simulink model "Ebike_Thermal_DT_v1"  (R2026a)
settings: configuration reference "VehicleVariable" (kept outside this file)
StartFcn:
  | %tic
StopFcn:
  | %toc
model workspace (MAT data in the model file):
  ExtDrvCmdsSwitch : Simulink.Parameter (value not decoded)
  ExtDrvRefSwitch : Simulink.Parameter (value not decoded)
  ExtEnvSwitch : Simulink.Parameter (value not decoded)
  ExtGndSwitch : Simulink.Parameter (value not decoded)
symbols that are objects in the model workspace (value not decoded): ExtDrvCmdsSwitch, ExtDrvRefSwitch, ExtEnvSwitch, ExtGndSwitch
undefined symbols (not defined in the file or in its folder): AmbTemp, BaroPress, CtrlTcuInitGear, CurvGradRef, CurvRef, DCM, DriverAeroRes, DriverDrivelineRes, DriverInitialGear, DriverPreviewDist, DriverRollRes, DriverShiftTime, DriverTimeConst, DriverTractiveForce, EnvAbsPrs, EnvAirTemp, EnvGrvty, EnvNomFrictionScaling, EnvNominalGrade, EnvScnFrictionMap, EnvScnFrictionMapXBpts, EnvScnFrictionMapYBpts, EnvScnHeightMap, EnvScnHeightMapXBpts, EnvScnHeightMapYBpts, EnvWindVelX, EnvWindVelY, EnvWindVelZ, Gnd, Grade, HazzardCmd, HighBeamCmd, lambda_mux, LeftSignalCmd, LngRef, LowBeamCmd, LtrRef, PhiRef, PlntThrCabRelHInit, PlntThrRefrigPinit, PlntVehDstCGRearAxl, PlntVehInitYawAng, PlntVehMass, PlntVehTrckWdth, PlntVehYawMomentInertia, PlntWhlLdRadiusFrnt, PlntWhlLdRadiusRear, PsiRef, RightSignalCmd, Sim3dSensor, Wind, XRef, YRef, Z
libraries: simulink x28, autolibutils x5, autolibsharedcommon x5, vehdynlibviscommon x4, vehdynlibdriver x2, sim3dgroundtruthsensorlib x2, autolibshared x2, sl3dlib x1, sharedtransform x1, sim3dlib x1
(part 5 of 5)

== system Ebike_Thermal_DT_v1/Environment/Varying Friction/Friction Map/2D Lookup Tbl for Scaling Fctr (Lambda) ==
  XWhl : Inport  Partition=on  PartitionDimension=1  PartitionWidth=1  PartitionOffset=0
  YWhl : Inport  Port=2  Partition=on  PartitionDimension=1  PartitionWidth=1  PartitionOffset=0
  2-D Lookup Table : Lookup_n-D  BreakpointsForDimension1=EnvScnFrictionMapXBpts  BreakpointsForDimension2=EnvScnFrictionMapYBpts  BeginIndexSearchUsingPreviousIndexResult=on  Table=EnvScnFrictionMap  InterpMethod=Nearest  ExtrapMethod=Clip  InternalRulePriority=Speed  RndMeth=Simplest
      settings: InputPortMap=u0,u1
  Add : Sum
  Add1 : Sum
  Constant : Constant  Value=0
  Constant1 : Constant  Value=0
  For Each : ForEach  DisableCoverage=on
  Unary Minus : UnaryMinus
  FricCoeffLambda : Outport  ConcatenationDimension=1
  wires:
  2-D Lookup Table/1 -> FricCoeffLambda/1
  YWhl/1 -> Unary Minus/1
  Constant1/1 -> Add1/1
  Constant/1 -> Add/2
  Add/1 -> 2-D Lookup Table/2
  Add1/1 -> 2-D Lookup Table/1
  Unary Minus/1 -> Add/1
  XWhl/1 -> Add1/2

== system Ebike_Thermal_DT_v1/Environment/Varying Friction/Friction Map/Wheel Coordinates ==
  FrntAxlLftX : Inport
  FrntAxlRghtX : Inport  Port=2
  RearAxlLftX : Inport  Port=3
  RearAxlRghtX : Inport  Port=4
  FrntAxlLftY : Inport  Port=5
  FrntAxlRghtY : Inport  Port=6
  RearAxlLftY : Inport  Port=7
  RearAxlRghtY : Inport  Port=8
  Matrix Concatenate : Concatenate  NumInputs=4  Mode=Multidimensional array
  Matrix Concatenate1 : Concatenate  NumInputs=4  Mode=Multidimensional array
  XWhl : Outport
  YWhl : Outport  Port=2
  wires:
  Matrix Concatenate1/1 -> YWhl/1
  FrntAxlLftX/1 -> Matrix Concatenate/1
  FrntAxlLftY/1 -> Matrix Concatenate1/1
  FrntAxlRghtY/1 -> Matrix Concatenate1/2
  FrntAxlRghtX/1 -> Matrix Concatenate/2
  RearAxlLftY/1 -> Matrix Concatenate1/3
  RearAxlLftX/1 -> Matrix Concatenate/3
  RearAxlRghtY/1 -> Matrix Concatenate1/4
  Matrix Concatenate/1 -> XWhl/1
  RearAxlRghtX/1 -> Matrix Concatenate/4

== system Ebike_Thermal_DT_v1/Environment/Varying Friction/Varying Friction/Road Track Friction ==
  XWhl : Inport
  YWhl : Inport  Port=2
  Cg : Inport  Port=3
  2D Lookup Tbl for Scaling Fctr (Lambda) : Subsystem  TreatAsAtomicUnit=on
      mask init:
      | [~]=vehdynicon('vehdynblk',gcb);
  Bus Selector : BusSelector  OutputSignals=X,Y
  Cnst Lambda : Constant  Value=ones(4,1).*lambda_g
  Constant1 : Constant  Value=SplitLambdaTrck
  Creating Inertial Frm Bpt : Subsystem
  En at t = 0 : Subsystem
  "Lambda (t = 0) " : Memory  InitialCondition=ones(4,1).*lambda_g  InheritSampleTime=on
  Switch : Switch  Criteria=u2 > Threshold  SaturateOnIntegerOverflow=off  InputSameDT=off
  FricCoeffLambda : Outport
  wires:
  YWhl/1 -> 2D Lookup Tbl for Scaling Fctr (Lambda)/2(YWhl)
  XWhl/1 -> 2D Lookup Tbl for Scaling Fctr (Lambda)/1(XWhl)
  2D Lookup Tbl for Scaling Fctr (Lambda)/1(Lambda for each whl) -> Switch/1
  "Lambda (t = 0) "/1 -> FricCoeffLambda/1
  Switch/1 -> "Lambda (t = 0) "/1
  Cnst Lambda/1 -> Switch/3
  Constant1/1 -> Switch/2
  Cg/1 -> Bus Selector/1
  Creating Inertial Frm Bpt/1(XBpt) -> 2D Lookup Tbl for Scaling Fctr (Lambda)/3(XBpt)
  Creating Inertial Frm Bpt/2(YBpt) -> 2D Lookup Tbl for Scaling Fctr (Lambda)/4(YBpt)
  Bus Selector/1 -> Creating Inertial Frm Bpt/1(XCg)  "<X>"
  Bus Selector/2 -> Creating Inertial Frm Bpt/2(YCg)  "<Y>"
  En at t = 0/1(Out1) -> Creating Inertial Frm Bpt/Enable

== system Ebike_Thermal_DT_v1/Environment/Varying Friction/Varying Friction/Wheel Coordinates ==
  FrntAxlLftX : Inport
  FrntAxlRghtX : Inport  Port=2
  RearAxlLftX : Inport  Port=3
  RearAxlRghtX : Inport  Port=4
  FrntAxlLftY : Inport  Port=5
  FrntAxlRghtY : Inport  Port=6
  RearAxlLftY : Inport  Port=7
  RearAxlRghtY : Inport  Port=8
  Matrix Concatenate : Concatenate  NumInputs=4  Mode=Multidimensional array
  Matrix Concatenate1 : Concatenate  NumInputs=4  Mode=Multidimensional array
  XWhl : Outport
  YWhl : Outport  Port=2
  wires:
  RearAxlRghtX/1 -> Matrix Concatenate/4
  Matrix Concatenate/1 -> XWhl/1
  RearAxlRghtY/1 -> Matrix Concatenate1/4
  RearAxlLftX/1 -> Matrix Concatenate/3
  RearAxlLftY/1 -> Matrix Concatenate1/3
  FrntAxlRghtX/1 -> Matrix Concatenate/2
  FrntAxlRghtY/1 -> Matrix Concatenate1/2
  FrntAxlLftY/1 -> Matrix Concatenate1/1
  FrntAxlLftX/1 -> Matrix Concatenate/1
  Matrix Concatenate1/1 -> YWhl/1

== system Ebike_Thermal_DT_v1/Visualization/Vehicle XY Plotter/XY View/Driveline Speed ==
  <EngSpd> : Inport
  <EMSpd> : Inport  Port=2
  Abs : Abs  ZeroCross=off  SaturateOnIntegerOverflow=off
  Abs1 : Abs  ZeroCross=off  SaturateOnIntegerOverflow=off
  Divide : Product  Inputs=*/
  Probe Dimension : Probe  ProbeWidth=off  ProbeSampleTime=off  ProbeComplexSignal=off  ProbeSignalDimensions=on
  Relational Operator : RelationalOperator  Operator=<=  OutDataTypeStr=boolean  ZeroCross=off  RndMeth=Simplest  InputSameDT=off
  Sum of Elements : Sum  Inputs=+
  Switch : Switch  Criteria=u2 > Threshold  ZeroCross=off  SaturateOnIntegerOverflow=off  InputSameDT=off
  MaxSpd : Outport
  wires:
  Switch/1 -> MaxSpd/1
  Sum of Elements/1 -> Divide/1
  Probe Dimension/1 -> Divide/2
  Divide/1 -> Switch/3, Abs1/1
  <EngSpd>/1 -> Switch/1, Abs/1
  Abs/1 -> Relational Operator/2
  <EMSpd>/1 -> Probe Dimension/1, Sum of Elements/1
  Relational Operator/1 -> Switch/2
  Abs1/1 -> Relational Operator/1

== system Ebike_Thermal_DT_v1/Visualization/Vehicle XY Plotter/XY View Ref/Driveline Speed ==
  <EngSpd> : Inport
  <EMSpd> : Inport  Port=2
  Abs : Abs  ZeroCross=off  SaturateOnIntegerOverflow=off
  Abs1 : Abs  ZeroCross=off  SaturateOnIntegerOverflow=off
  Divide : Product  Inputs=*/
  Probe Dimension : Probe  ProbeWidth=off  ProbeSampleTime=off  ProbeComplexSignal=off  ProbeSignalDimensions=on
  Relational Operator : RelationalOperator  Operator=<=  OutDataTypeStr=boolean  ZeroCross=off  RndMeth=Simplest  InputSameDT=off
  Sum of Elements : Sum  Inputs=+
  Switch : Switch  Criteria=u2 > Threshold  ZeroCross=off  SaturateOnIntegerOverflow=off  InputSameDT=off
  MaxSpd : Outport
  wires:
  Switch/1 -> MaxSpd/1
  Sum of Elements/1 -> Divide/1
  Probe Dimension/1 -> Divide/2
  Divide/1 -> Switch/3, Abs1/1
  <EngSpd>/1 -> Switch/1, Abs/1
  Abs/1 -> Relational Operator/2
  <EMSpd>/1 -> Probe Dimension/1, Sum of Elements/1
  Relational Operator/1 -> Switch/2
  Abs1/1 -> Relational Operator/1

== system Ebike_Thermal_DT_v1/Visualization/Vehicle XY Plotter/XY View Ref with One-Axle Trailer/Driveline Speed ==
  <EngSpd> : Inport
  <EMSpd> : Inport  Port=2
  Abs : Abs  ZeroCross=off  SaturateOnIntegerOverflow=off
  Abs1 : Abs  ZeroCross=off  SaturateOnIntegerOverflow=off
  Divide : Product  Inputs=*/
  Probe Dimension : Probe  ProbeWidth=off  ProbeSampleTime=off  ProbeComplexSignal=off  ProbeSignalDimensions=on
  Relational Operator : RelationalOperator  Operator=<=  OutDataTypeStr=boolean  ZeroCross=off  RndMeth=Simplest  InputSameDT=off
  Sum of Elements : Sum  Inputs=+
  Switch : Switch  Criteria=u2 > Threshold  ZeroCross=off  SaturateOnIntegerOverflow=off  InputSameDT=off
  MaxSpd : Outport
  wires:
  Switch/1 -> MaxSpd/1
  Sum of Elements/1 -> Divide/1
  Probe Dimension/1 -> Divide/2
  Divide/1 -> Switch/3, Abs1/1
  <EngSpd>/1 -> Switch/1, Abs/1
  Abs/1 -> Relational Operator/2
  <EMSpd>/1 -> Probe Dimension/1, Sum of Elements/1
  Relational Operator/1 -> Switch/2
  Abs1/1 -> Relational Operator/1

== system Ebike_Thermal_DT_v1/Driver Commands/Driver Commands/Longitudinal Driver/Hill Hold & Stop/Hill Hold ==
  <EngSpdOut> : Inport
  <xdot> : Inport  Port=2
  <BattSoc> : Inport  Port=3
  LngRef : Inport  Port=4
  <Grade> : Inport  Port=5
  Abs : Abs  ZeroCross=off  SaturateOnIntegerOverflow=off
  Abs1 : Abs  ZeroCross=off  SaturateOnIntegerOverflow=off
  Compare To Constant : simulink/Logic and Bit Operations/Compare To Constant  relop=<=  const=.1  OutDataTypeStr=boolean  ZeroCross=off
  Compare To Constant1 : simulink/Logic and Bit Operations/Compare To Constant  relop=>=  const=.1  OutDataTypeStr=boolean  ZeroCross=off
  Compare To Constant2 : simulink/Logic and Bit Operations/Compare To Constant  relop=<=  const=500  OutDataTypeStr=boolean  ZeroCross=off
  Compare To Constant3 : simulink/Logic and Bit Operations/Compare To Constant  relop=<=  const=5  OutDataTypeStr=boolean  ZeroCross=off
  Compare To Constant4 : simulink/Logic and Bit Operations/Compare To Constant  relop=<=  const=.1  OutDataTypeStr=boolean  ZeroCross=off
  Data Type Conversion1 : DataTypeConversion  SaturateOnIntegerOverflow=off  RndMeth=Floor
  Logical Operator : Logic  AllPortsSameDT=off  OutDataTypeStr=boolean
  Logical Operator1 : Logic  Inputs=3  AllPortsSameDT=off  OutDataTypeStr=boolean
  Logical Operator2 : Logic  Operator=OR  AllPortsSameDT=off  OutDataTypeStr=boolean
  Signal Specification : SignalSpecification  Unit=m/s
  Unit Conversion : UnitConversion
  DecelOvr : Outport
  EnblDecelOvr : Outport  Port=2
  wires:
  <BattSoc>/1 -> Compare To Constant4/1
  <xdot>/1 -> Unit Conversion/1
  <Grade>/1 -> Abs1/1
  Compare To Constant4/1 -> Logical Operator1/3
  <EngSpdOut>/1 -> Compare To Constant2/1
  Signal Specification/1 -> Compare To Constant3/1
  Abs/1 -> Compare To Constant/1
  Logical Operator1/1 -> Logical Operator2/1
  Data Type Conversion1/1 -> EnblDecelOvr/1
  Compare To Constant2/1 -> Logical Operator1/1
  Logical Operator/1 -> Logical Operator2/2
  Compare To Constant3/1 -> Logical Operator1/2
  Compare To Constant1/1 -> Logical Operator/2
  LngRef/1 -> Abs/1
  Abs1/1 -> Compare To Constant1/1
  Logical Operator2/1 -> Data Type Conversion1/1, DecelOvr/1
  Unit Conversion/1 -> Signal Specification/1
  Compare To Constant/1 -> Logical Operator/1

== system Ebike_Thermal_DT_v1/Driver Commands/Driver Commands/Longitudinal Driver/Hill Hold & Stop/Stop Detection ==
  LngRef : Inport
  <xdot> : Inport  Port=2
  Abs2 : Abs  ZeroCross=off  SaturateOnIntegerOverflow=off
  Compare To Constant5 : simulink/Logic and Bit Operations/Compare To Constant  relop=<=  const=.1  OutDataTypeStr=boolean  ZeroCross=off
  Compare To Constant6 : simulink/Logic and Bit Operations/Compare To Constant  relop===  const=0  OutDataTypeStr=boolean  ZeroCross=off
  Data Type Conversion2 : DataTypeConversion  SaturateOnIntegerOverflow=off  RndMeth=Floor
  Gain : Gain  Gain=.1
  LatchSwitchCont : autolibutils/LatchSwitchCont  aMode=6
  Logical Operator1 : Logic  Operator=NOT  AllPortsSameDT=off  OutDataTypeStr=boolean
  Logical Operator3 : Logic  AllPortsSameDT=off  OutDataTypeStr=boolean
  DecelOvrCmd : Outport
  EnblDecelOvr : Outport  Port=2
  wires:
  <xdot>/1 -> Abs2/1
  Gain/1 -> DecelOvrCmd/1
  Compare To Constant6/1 -> Logical Operator3/2, Logical Operator1/1
  Logical Operator1/1 -> LatchSwitchCont/2
  Data Type Conversion2/1 -> Gain/1
  LatchSwitchCont/1 -> Data Type Conversion2/1, EnblDecelOvr/1
  Abs2/1 -> Compare To Constant5/1
  LngRef/1 -> Compare To Constant6/1
  Logical Operator3/1 -> LatchSwitchCont/1
  Compare To Constant5/1 -> Logical Operator3/1

== system Ebike_Thermal_DT_v1/Driver Commands/Driver Commands/Longitudinal Driver/Longitudinal Driver/External Action Routing ==
  EnblAccelOvr : Inport  OutDataTypeStr=boolean  Unit=1  PortDimensions=1
  AccelOvrCmd : Inport  Port=2  OutDataTypeStr=double  Unit=1  PortDimensions=1
  AccelHld : Inport  Port=3  OutDataTypeStr=boolean  Unit=1  PortDimensions=1
  AccelZero : Inport  Port=4  OutDataTypeStr=boolean  Unit=1  PortDimensions=1
  EnblDecelOvr : Inport  Port=5  OutDataTypeStr=boolean  Unit=1  PortDimensions=1
  DecelOvrCmd : Inport  Port=6  OutDataTypeStr=double  Unit=1  PortDimensions=1
  DecelHld : Inport  Port=7  OutDataTypeStr=boolean  Unit=1  PortDimensions=1
  DecelZero : Inport  Port=8  OutDataTypeStr=boolean  Unit=1  PortDimensions=1
  Bus Creator2 : BusCreator  Inputs=8
  ExtActions : Outport
  wires:
  Bus Creator2/1 -> ExtActions/1  "ExtActions"
  DecelZero/1 -> Bus Creator2/8  "DecelZero"
  DecelHld/1 -> Bus Creator2/7  "DecelHld"
  DecelOvrCmd/1 -> Bus Creator2/6  "DecelOvrCmd"
  EnblDecelOvr/1 -> Bus Creator2/5  "EnblDecelOvr"
  AccelZero/1 -> Bus Creator2/4  "AccelZero"
  AccelHld/1 -> Bus Creator2/3  "AccelHld"
  AccelOvrCmd/1 -> Bus Creator2/2  "AccelOvrCmd"
  EnblAccelOvr/1 -> Bus Creator2/1  "EnblAccelOvr"

== system Ebike_Thermal_DT_v1/Driver Commands/Driver Commands/Predictive Driver/Hill Hold & Stop/Hill Hold ==
  <EngSpdOut> : Inport
  <xdot> : Inport  Port=2
  <BattSoc> : Inport  Port=3
  LngRef : Inport  Port=4
  <Grade> : Inport  Port=5
  Abs : Abs  ZeroCross=off  SaturateOnIntegerOverflow=off
  Abs1 : Abs  ZeroCross=off  SaturateOnIntegerOverflow=off
  Compare To Constant : simulink/Logic and Bit Operations/Compare To Constant  relop=<=  const=.1  OutDataTypeStr=boolean  ZeroCross=off
  Compare To Constant1 : simulink/Logic and Bit Operations/Compare To Constant  relop=>=  const=.1  OutDataTypeStr=boolean  ZeroCross=off
  Compare To Constant2 : simulink/Logic and Bit Operations/Compare To Constant  relop=<=  const=500  OutDataTypeStr=boolean  ZeroCross=off
  Compare To Constant3 : simulink/Logic and Bit Operations/Compare To Constant  relop=<=  const=5  OutDataTypeStr=boolean  ZeroCross=off
  Compare To Constant4 : simulink/Logic and Bit Operations/Compare To Constant  relop=<=  const=.1  OutDataTypeStr=boolean  ZeroCross=off
  Data Type Conversion1 : DataTypeConversion  SaturateOnIntegerOverflow=off  RndMeth=Floor
  Logical Operator : Logic  AllPortsSameDT=off  OutDataTypeStr=boolean
  Logical Operator1 : Logic  Inputs=3  AllPortsSameDT=off  OutDataTypeStr=boolean
  Logical Operator2 : Logic  Operator=OR  AllPortsSameDT=off  OutDataTypeStr=boolean
  Signal Specification : SignalSpecification  Unit=m/s
  Unit Conversion : UnitConversion
  DecelOvr : Outport
  EnblDecelOvr : Outport  Port=2
  wires:
  <BattSoc>/1 -> Compare To Constant4/1
  <xdot>/1 -> Unit Conversion/1
  <Grade>/1 -> Abs1/1
  Compare To Constant4/1 -> Logical Operator1/3
  <EngSpdOut>/1 -> Compare To Constant2/1
  Signal Specification/1 -> Compare To Constant3/1
  Abs/1 -> Compare To Constant/1
  Logical Operator1/1 -> Logical Operator2/1
  Data Type Conversion1/1 -> EnblDecelOvr/1
  Compare To Constant2/1 -> Logical Operator1/1
  Logical Operator/1 -> Logical Operator2/2
  Compare To Constant3/1 -> Logical Operator1/2
  Compare To Constant1/1 -> Logical Operator/2
  LngRef/1 -> Abs/1
  Abs1/1 -> Compare To Constant1/1
  Logical Operator2/1 -> Data Type Conversion1/1, DecelOvr/1
  Unit Conversion/1 -> Signal Specification/1
  Compare To Constant/1 -> Logical Operator/1

== system Ebike_Thermal_DT_v1/Driver Commands/Driver Commands/Predictive Driver/Hill Hold & Stop/Stop Detection ==
  LngRef : Inport
  <xdot> : Inport  Port=2
  Abs2 : Abs  ZeroCross=off  SaturateOnIntegerOverflow=off
  Compare To Constant5 : simulink/Logic and Bit Operations/Compare To Constant  relop=<=  const=.1  OutDataTypeStr=boolean  ZeroCross=off
  Compare To Constant6 : simulink/Logic and Bit Operations/Compare To Constant  relop===  const=0  OutDataTypeStr=boolean  ZeroCross=off
  Data Type Conversion2 : DataTypeConversion  SaturateOnIntegerOverflow=off  RndMeth=Floor
  Gain : Gain  Gain=.1
  LatchSwitchCont : autolibutils/LatchSwitchCont  aMode=6
  Logical Operator1 : Logic  Operator=NOT  AllPortsSameDT=off  OutDataTypeStr=boolean
  Logical Operator3 : Logic  AllPortsSameDT=off  OutDataTypeStr=boolean
  DecelOvrCmd : Outport
  EnblDecelOvr : Outport  Port=2
  wires:
  <xdot>/1 -> Abs2/1
  Gain/1 -> DecelOvrCmd/1
  Compare To Constant6/1 -> Logical Operator3/2, Logical Operator1/1
  Logical Operator1/1 -> LatchSwitchCont/2
  Data Type Conversion2/1 -> Gain/1
  LatchSwitchCont/1 -> Data Type Conversion2/1, EnblDecelOvr/1
  Abs2/1 -> Compare To Constant5/1
  LngRef/1 -> Compare To Constant6/1
  Logical Operator3/1 -> LatchSwitchCont/1
  Compare To Constant5/1 -> Logical Operator3/1

== system Ebike_Thermal_DT_v1/Driver Commands/Driver Commands/Predictive Stanley Driver/Hill Hold & Stop/Hill Hold ==
  <EngSpdOut> : Inport
  <xdot> : Inport  Port=2
  <BattSoc> : Inport  Port=3
  LngRef : Inport  Port=4
  <Grade> : Inport  Port=5
  Abs : Abs  ZeroCross=off  SaturateOnIntegerOverflow=off
  Abs1 : Abs  ZeroCross=off  SaturateOnIntegerOverflow=off
  Compare To Constant : simulink/Logic and Bit Operations/Compare To Constant  relop=<=  const=.1  OutDataTypeStr=boolean  ZeroCross=off
  Compare To Constant1 : simulink/Logic and Bit Operations/Compare To Constant  relop=>=  const=.1  OutDataTypeStr=boolean  ZeroCross=off
  Compare To Constant2 : simulink/Logic and Bit Operations/Compare To Constant  relop=<=  const=500  OutDataTypeStr=boolean  ZeroCross=off
  Compare To Constant3 : simulink/Logic and Bit Operations/Compare To Constant  relop=<=  const=5  OutDataTypeStr=boolean  ZeroCross=off
  Compare To Constant4 : simulink/Logic and Bit Operations/Compare To Constant  relop=<=  const=.1  OutDataTypeStr=boolean  ZeroCross=off
  Data Type Conversion1 : DataTypeConversion  SaturateOnIntegerOverflow=off  RndMeth=Floor
  Logical Operator : Logic  AllPortsSameDT=off  OutDataTypeStr=boolean
  Logical Operator1 : Logic  Inputs=3  AllPortsSameDT=off  OutDataTypeStr=boolean
  Logical Operator2 : Logic  Operator=OR  AllPortsSameDT=off  OutDataTypeStr=boolean
  Signal Specification : SignalSpecification  Unit=m/s
  Unit Conversion : UnitConversion
  DecelOvr : Outport
  EnblDecelOvr : Outport  Port=2
  wires:
  <BattSoc>/1 -> Compare To Constant4/1
  <xdot>/1 -> Unit Conversion/1
  <Grade>/1 -> Abs1/1
  Compare To Constant4/1 -> Logical Operator1/3
  <EngSpdOut>/1 -> Compare To Constant2/1
  Signal Specification/1 -> Compare To Constant3/1
  Abs/1 -> Compare To Constant/1
  Logical Operator1/1 -> Logical Operator2/1
  Data Type Conversion1/1 -> EnblDecelOvr/1
  Compare To Constant2/1 -> Logical Operator1/1
  Logical Operator/1 -> Logical Operator2/2
  Compare To Constant3/1 -> Logical Operator1/2
  Compare To Constant1/1 -> Logical Operator/2
  LngRef/1 -> Abs/1
  Abs1/1 -> Compare To Constant1/1
  Logical Operator2/1 -> Data Type Conversion1/1, DecelOvr/1
  Unit Conversion/1 -> Signal Specification/1
  Compare To Constant/1 -> Logical Operator/1

== system Ebike_Thermal_DT_v1/Driver Commands/Driver Commands/Predictive Stanley Driver/Hill Hold & Stop/Stop Detection ==
  LngRef : Inport
  <xdot> : Inport  Port=2
  Abs2 : Abs  ZeroCross=off  SaturateOnIntegerOverflow=off
  Compare To Constant5 : simulink/Logic and Bit Operations/Compare To Constant  relop=<=  const=.1  OutDataTypeStr=boolean  ZeroCross=off
  Compare To Constant6 : simulink/Logic and Bit Operations/Compare To Constant  relop===  const=0  OutDataTypeStr=boolean  ZeroCross=off
  Data Type Conversion2 : DataTypeConversion  SaturateOnIntegerOverflow=off  RndMeth=Floor
  Gain : Gain  Gain=.1
  LatchSwitchCont : autolibutils/LatchSwitchCont  aMode=6
  Logical Operator1 : Logic  Operator=NOT  AllPortsSameDT=off  OutDataTypeStr=boolean
  Logical Operator3 : Logic  AllPortsSameDT=off  OutDataTypeStr=boolean
  DecelOvrCmd : Outport
  EnblDecelOvr : Outport  Port=2
  wires:
  <xdot>/1 -> Abs2/1
  Gain/1 -> DecelOvrCmd/1
  Compare To Constant6/1 -> Logical Operator3/2, Logical Operator1/1
  Logical Operator1/1 -> LatchSwitchCont/2
  Data Type Conversion2/1 -> Gain/1
  LatchSwitchCont/1 -> Data Type Conversion2/1, EnblDecelOvr/1
  Abs2/1 -> Compare To Constant5/1
  LngRef/1 -> Compare To Constant6/1
  Logical Operator3/1 -> LatchSwitchCont/1
  Compare To Constant5/1 -> Logical Operator3/1

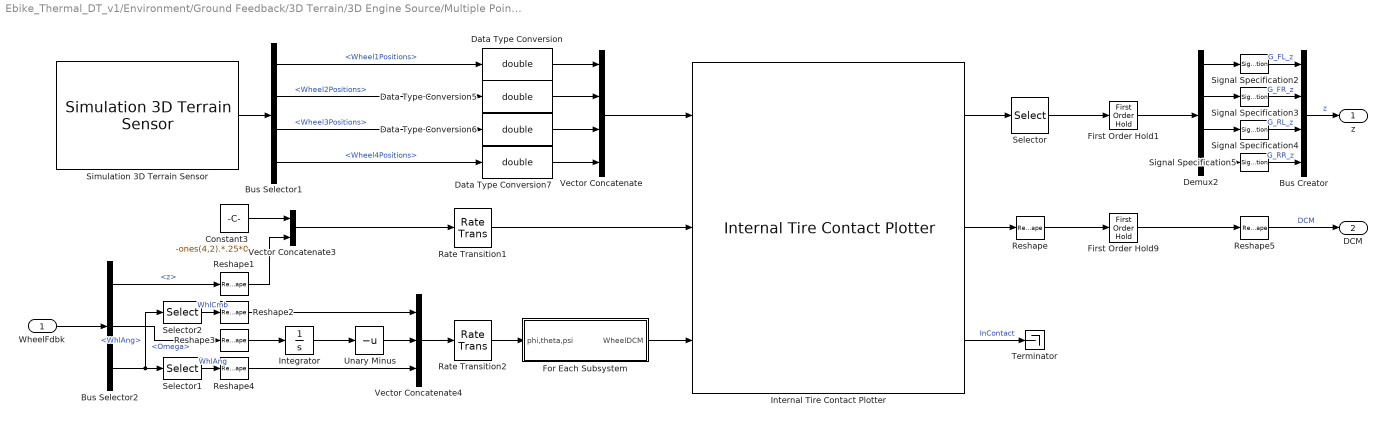
== system Ebike_Thermal_DT_v1/Environment/Ground Feedback/3D Terrain/3D Engine Source/Multiple Points ==
  WheelFdbk : Inport
  Bus Creator : BusCreator  Inputs=4
  Bus Selector1 : BusSelector  OutputSignals=Wheel1Positions,Wheel2Positions,Wheel3Positions,Wheel4Positions
  Bus Selector2 : BusSelector  OutputSignals=z,Omega,WhlAng
  Constant3 : Constant  Value=-ones(4,2).*.25*0
  Data Type Conversion{,5..7} (4 alike) : DataTypeConversion  OutDataTypeStr=double  SaturateOnIntegerOverflow=off  RndMeth=Floor
  Demux2 : Demux
  First Order Hold1 : FirstOrderHold  OutputAlgorithm=Fast (Minimize Error)  ErrorTolerance=.001
  First Order Hold9 : FirstOrderHold  InitialOutput=reshape(repmat(eye(3),1,1,4),[],1)  OutputAlgorithm=Fast (Minimize Error)  ErrorTolerance=.001
  For Each Subsystem : Subsystem  TreatAsAtomicUnit=on
  Integrator : Integrator  WrapState=on  ZeroCross=off
  Internal Tire Contact Plotter : vehdynlibviscommon/Internal Tire Contact Plotter  dispFig=off  numAxles=2  numWheelsPerAxle=2  wheelRad=.33  wheelWidth=.235  rayOrigins=[0.5 -0.5 0;0.4 -0.5 0;0.3 -0.5 0;0.19999999999999996 -0.5 0;0.099999999999999978 -0.5 0;0 -0.5 0;-0.099999999999999978 -0.5 0;-0.19999999999999996 -0.5 0;-0.3 -0.5 0;-0.4 -0.5 0;-0.5 -0.5 0;0.5 -0.4 0;0.4 -0.4 0;0.3 -0.4 0;0.19999999999999996 -0.4 0;0.099999999999999978 -0.4 0;0 -0.4 0;-0.099999999999999978 -0.4 0;-0.19999999999999996 -0.4 0;-0.3 -0.4 0;-0.4 -0.4 0;-0.5 -0.4 0;0.5 -0.3 0;0.4 -0.3 0;0.3 -0.3 0;0.19999999999999996 -0.3 0;0.099999999999999978 -0.3 0;0 -0.3 0;-0.099999999999999978 -0.3 0;-0.19999999999999996 -0.3 0;-0.3 -0.3 0;-0.4 -0.3 0;-0.5 -0.3 0;0.5 -0.19999999999999996 0;0.4 -0.19999999999999996 0;0.3 -0.19999999999999996 0;0.19999999999999996 -0.19999999999999996 0;0.099999999999999978 -0.19999999999999996 0;0 -0.19999999999999996 0;-0.099999999999999978 -0.19999999999999996 0;-0.19999999999999996 -0.19999999999999996 0;-0.3 -0.19999999999999996 0;-0.4 -0.19999999999999996 0;-0.5 -0.19999999999999996 0;0.5 -0.099999999999999978 0;0.4 -0.099999999999999978 0;0.3 -0.099999999999999978 0;0.19999999999999996 -0.099999999999999978 0;0.099999999999999978 -0.099999999999999978 0;0 -0.099999999999999978 0;-0.099999999999999978 -0.099999999999999978 0;-0.19999999999999996 -0.099999999999999978 0;-0.3 -0.099999999999999978 0;-0.4 -0.099999999999999978 0;-0.5 -0.099999999999999978 0;0.5 0 0;0.4 0 0;0.3 0 0;0.19999999999999996 0 0;0.099999999999999978 0 0;0 0 0;-0.099999999999999978 0 0;-0.19999999999999996 0 0;-0.3 0 0;-0.4 0 0;-0.5 0 0;0.5 0.099999999999999978 0;0.4 0.099999999999999978 0;0.3 0.099999999999999978 0;0.19999999999999996 0.099999999999999978 0;0.099999999999999978 0.099999999999999978 0;0 0.099999999999999978 0;-0.099999999999999978 0.099999999999999978 0;-0.19999999999999996 0.099999999999999978 0;-0.3 0.099999999999999978 0;-0.4 0.099999999999999978 0;-0.5 0.099999999999999978 0;0.5 0.19999999999999996 0;0.4 0.19999999999999996 0;0.3 0.19999999999999996 0;0.19999999999999996 0.19999999999999996 0;0.099999999999999978 0.19999999999999996 0;0 0.19999999999999996 0;-0.099999999999999978 0.19999999999999996 0;-0.19999999999999996 0.19999999999999996 0;-0.3 0.19999999999999996 0;-0.4 0.19999999999999996 0;-0.5 0.19999999999999996 0;0.5 0.3 0;0.4 0.3 0;0.3 0.3 0;0.19999999999999996 0.3 0;0.099999999999999978 0.3 0;0 0.3 0;-0.099999999999999978 0.3 0;-0.19999999999999996 0.3 0;-0.3 0.3 0;-0.4 0.3 0;-0.5 0.3 0;0.5 0.4 0;0.4 0.4 0;0.3 0.4 0;0.19999999999999996 0.4 0;0.099999999999999978 0.4 0;0 0.4 0;-0.099999999999999978 0.4 0;-0.19999999999999996 0.4 0;-0.3 0.4 0;-0.4 0.4 0;-0.5 0.4 0;0.5 0.5 0;0.4 0.5 0;0.3 0.5 0;0.19999999999999996 0.5 0;0.099999999999999978 0.5 0;0 0.5 0;-0.099999999999999978 0.5 0;-0.19999999999999996 0.5 0;-0.3 0.5 0;-0.4 0.5 0;-0.5 0.5 0]
  Rate Transition1 : RateTransition  Integrity=off  Deterministic=off  OutPortSampleTime=.01
  Rate Transition2 : RateTransition  Integrity=off  Deterministic=off  OutPortSampleTime=.01
  Reshape : Reshape  OutputDimensionality=Column vector (2-D)
  Reshape1 : Reshape  OutputDimensionality=Column vector (2-D)
  Reshape2 : Reshape  OutputDimensionality=Row vector (2-D)
  Reshape3 : Reshape  OutputDimensionality=Row vector (2-D)
  Reshape4 : Reshape  OutputDimensionality=Row vector (2-D)
  Reshape5 : Reshape  OutputDimensionality=Customize  OutputDimensions=[3,3,4]
  Selector : Selector  NumberOfDimensions=2  InputPortWidth=3  IndexOptions=Select all,Index vector (dialog)  Indices=[1 3],3  OutputSizes=1,1
  Selector1 : Selector  NumberOfDimensions=2  InputPortWidth=3  IndexOptions=Index vector (dialog),Select all  Indices=[3],1  OutputSizes=1,1
  Selector2 : Selector  NumberOfDimensions=2  InputPortWidth=3  IndexOptions=Index vector (dialog),Select all  Indices=[1],1  OutputSizes=1,1
  Signal Specification{2..5} (4 alike) : SignalSpecification  Unit=m
  Simulation 3D Terrain Sensor : sim3dgroundtruthsensorlib/Simulation 3D Terrain Sensor  Priority=1  vehTagList={'Scene Origin';'SimulinkVehicle1';'0'}  sensorTag=Sim3dSensor�  sensorId=1  sensorName=Sim3dSensor�  vehTag=SimulinkVehicle1  CoordinateSystem=Default  tmountOffset=[0, 0, 0]  rmountOffset=[0,0,0,]  RayOrigins=[0.5 -0.5 0;0.4 -0.5 0;0.3 -0.5 0;0.19999999999999996 -0.5 0;0.099999999999999978 -0.5 0;0 -0.5 0;-0.099999999999999978 -0.5 0;-0.19999999999999996 -0.5 0;-0.3 -0.5 0;-0.4 -0.5 0;-0.5 -0.5 0;0.5 -0.4 0;0.4 -0.4 0;0.3 -0.4 0;0.19999999999999996 -0.4 0;0.099999999999999978 -0.4 0;0 -0.4 0;-0.099999999999999978 -0.4 0;-0.19999999999999996 -0.4 0;-0.3 -0.4 0;-0.4 -0.4 0;-0.5 -0.4 0;0.5 -0.3 0;0.4 -0.3 0;0.3 -0.3 0;0.19999999999999996 -0.3 0;0.099999999999999978 -0.3 0;0 -0.3 0;-0.099999999999999978 -0.3 0;-0.19999999999999996 -0.3 0;-0.3 -0.3 0;-0.4 -0.3 0;-0.5 -0.3 0;0.5 -0.19999999999999996 0;0.4 -0.19999999999999996 0;0.3 -0.19999999999999996 0;0.19999999999999996 -0.19999999999999996 0;0.099999999999999978 -0.19999999999999996 0;0 -0.19999999999999996 0;-0.099999999999999978 -0.19999999999999996 0;-0.19999999999999996 -0.19999999999999996 0;-0.3 -0.19999999999999996 0;-0.4 -0.19999999999999996 0;-0.5 -0.19999999999999996 0;0.5 -0.099999999999999978 0;0.4 -0.099999999999999978 0;0.3 -0.099999999999999978 0;0.19999999999999996 -0.099999999999999978 0;0.099999999999999978 -0.099999999999999978 0;0 -0.099999999999999978 0;-0.099999999999999978 -0.099999999999999978 0;-0.19999999999999996 -0.099999999999999978 0;-0.3 -0.099999999999999978 0;-0.4 -0.099999999999999978 0;-0.5 -0.099999999999999978 0;0.5 0 0;0.4 0 0;0.3 0 0;0.19999999999999996 0 0;0.099999999999999978 0 0;0 0 0;-0.099999999999999978 0 0;-0.19999999999999996 0 0;-0.3 0 0;-0.4 0 0;-0.5 0 0;0.5 0.099999999999999978 0;0.4 0.099999999999999978 0;0.3 0.099999999999999978 0;0.19999999999999996 0.099999999999999978 0;0.099999999999999978 0.099999999999999978 0;0 0.099999999999999978 0;-0.099999999999999978 0.099999999999999978 0;-0.19999999999999996 0.099999999999999978 0;-0.3 0.099999999999999978 0;-0.4 0.099999999999999978 0;-0.5 0.099999999999999978 0;0.5 0.19999999999999996 0;0.4 0.19999999999999996 0;0.3 0.19999999999999996 0;0.19999999999999996 0.19999999999999996 0;0.099999999999999978 0.19999999999999996 0;0 0.19999999999999996 0;-0.099999999999999978 0.19999999999999996 0;-0.19999999999999996 0.19999999999999996 0;-0.3 0.19999999999999996 0;-0.4 0.19999999999999996 0;-0.5 0.19999999999999996 0;0.5 0.3 0;0.4 0.3 0;0.3 0.3 0;0.19999999999999996 0.3 0;0.099999999999999978 0.3 0;0 0.3 0;-0.099999999999999978 0.3 0;-0.19999999999999996 0.3 0;-0.3 0.3 0;-0.4 0.3 0;-0.5 0.3 0;0.5 0.4 0;0.4 0.4 0;0.3 0.4 0;0.19999999999999996 0.4 0;0.099999999999999978 0.4 0;0 0.4 0;-0.099999999999999978 0.4 0;-0.19999999999999996 0.4 0;-0.3 0.4 0;-0.4 0.4 0;-0.5 0.4 0;0.5 0.5 0;0.4 0.5 0;0.3 0.5 0;0.19999999999999996 0.5 0;0.099999999999999978 0.5 0;0 0.5 0;-0.099999999999999978 0.5 0;-0.19999999999999996 0.5 0;-0.3 0.5 0;-0.4 0.5 0;-0.5 0.5 0]  RayDirections=[0 0 -1;0 0 -1;0 0 -1;0 0 -1;0 0 -1;0 0 -1;0 0 -1;0 0 -1;0 0 -1;0 0 -1;0 0 -1;0 0 -1;0 0 -1;0 0 -1;0 0 -1;0 0 -1;0 0 -1;0 0 -1;0 0 -1;0 0 -1;0 0 -1;0 0 -1;0 0 -1;0 0 -1;0 0 -1;0 0 -1;0 0 -1;0 0 -1;0 0 -1;0 0 -1;0 0 -1;0 0 -1;0 0 -1;0 0 -1;0 0 -1;0 0 -1;0 0 -1;0 0 -1;0 0 -1;0 0 -1;0 0 -1;0 0 -1;0 0 -1;0 0 -1;0 0 -1;0 0 -1;0 0 -1;0 0 -1;0 0 -1;0 0 -1;0 0 -1;0 0 -1;0 0 -1;0 0 -1;0 0 -1;0 0 -1;0 0 -1;0 0 -1;0 0 -1;0 0 -1;0 0 -1;0 0 -1;0 0 -1;0 0 -1;0 0 -1;0 0 -1;0 0 -1;0 0 -1;0 0 -1;0 0 -1;0 0 -1;0 0 -1;0 0 -1;0 0 -1;0 0 -1;0 0 -1;0 0 -1;0 0 -1;0 0 -1;0 0 -1;0 0 -1;0 0 -1;0 0 -1;0 0 -1;0 0 -1;0 0 -1;0 0 -1;0 0 -1;0 0 -1;0 0 -1;0 0 -1;0 0 -1;0 0 -1;0 0 -1;0 0 -1;0 0 -1;0 0 -1;0 0 -1;0 0 -1;0 0 -1;0 0 -1;0 0 -1;0 0 -1;0 0 -1;0 0 -1;0 0 -1;0 0 -1;0 0 -1;0 0 -1;0 0 -1;0 0 -1;0 0 -1;0 0 -1;0 0 -1;0 0 -1;0 0 -1;0 0 -1;0 0 -1;0 0 -1;0 0 -1;0 0 -1]  RayLengths=[20;20;20;20;20;20;20;20;20;20;20;20;20;20;20;20;20;20;20;20;20;20;20;20;20;20;20;20;20;20;20;20;20;20;20;20;20;20;20;20;20;20;20;20;20;20;20;20;20;20;20;20;20;20;20;20;20;20;20;20;20;20;20;20;20;20;20;20;20;20;20;20;20;20;20;20;20;20;20;20;20;20;20;20;20;20;20;20;20;20;20;20;20;20;20;20;20;20;20;20;20;20;20;20;20;20;20;20;20;20;20;20;20;20;20;20;20;20;20;20;20]  NumberOfWheels=4  VisualizeTraceLines=off  SampleTime=-1  aMode=2  ID=1
  Terminator : Terminator
  Unary Minus : UnaryMinus
  Vector Concatenate : Concatenate  NumInputs=4  Mode=Multidimensional array  ConcatenateDimension=3
  Vector Concatenate3 : Concatenate  Mode=Multidimensional array  ConcatenateDimension=2
  Vector Concatenate4 : Concatenate  NumInputs=3  Mode=Multidimensional array
  z : Outport
  DCM : Outport  Port=2
  wires:
  Data Type Conversion6/1 -> Vector Concatenate/3
  Selector/1 -> First Order Hold1/1
  Signal Specification5/1 -> Bus Creator/4  "G_RR_z"
  Bus Selector1/3 -> Data Type Conversion6/1  "<Wheel3Positions>"
  Demux2/2 -> Signal Specification3/1
  Data Type Conversion/1 -> Vector Concatenate/1
  Data Type Conversion5/1 -> Vector Concatenate/2
  Demux2/3 -> Signal Specification4/1
  Internal Tire Contact Plotter/1 -> Selector/1
  Internal Tire Contact Plotter/3 -> Terminator/1  "InContact"
  Vector Concatenate/1 -> Internal Tire Contact Plotter/1
  Data Type Conversion7/1 -> Vector Concatenate/4
  Bus Selector1/1 -> Data Type Conversion/1  "<Wheel1Positions>"
  Demux2/4 -> Signal Specification5/1
  Bus Creator/1 -> z/1  "z"
  Signal Specification2/1 -> Bus Creator/1  "G_FL_z"
  Bus Selector1/4 -> Data Type Conversion7/1  "<Wheel4Positions>"
  Signal Specification3/1 -> Bus Creator/2  "G_FR_z"
  Signal Specification4/1 -> Bus Creator/3  "G_RL_z"
  Bus Selector1/2 -> Data Type Conversion5/1  "<Wheel2Positions>"
  Demux2/1 -> Signal Specification2/1
  Simulation 3D Terrain Sensor/1 -> Bus Selector1/1
  Reshape5/1 -> DCM/1  "DCM"
  Internal Tire Contact Plotter/2 -> Reshape/1
  Integrator/1 -> Unary Minus/1
  Bus Selector2/2 -> Reshape3/1  "<Omega>"
  Vector Concatenate3/1 -> Rate Transition1/1
  For Each Subsystem/1(WheelDCM) -> Internal Tire Contact Plotter/3
  Reshape3/1 -> Integrator/1
  Vector Concatenate4/1 -> Rate Transition2/1
  Reshape4/1 -> Vector Concatenate4/3
  Rate Transition2/1 -> For Each Subsystem/1(phi,theta,psi)
  Reshape1/1 -> Vector Concatenate3/2
  WheelFdbk/1 -> Bus Selector2/1
  Bus Selector2/1 -> Reshape1/1  "<z>"
  Bus Selector2/3 -> Selector2/1, Selector1/1  "<WhlAng>"
  Constant3/1 -> Vector Concatenate3/1
  Reshape2/1 -> Vector Concatenate4/1
  Unary Minus/1 -> Vector Concatenate4/2
  Rate Transition1/1 -> Internal Tire Contact Plotter/2
  First Order Hold9/1 -> Reshape5/1
  Reshape/1 -> First Order Hold9/1
  First Order Hold1/1 -> Demux2/1
  Selector1/1 -> Reshape4/1  "WhlAng"
  Selector2/1 -> Reshape2/1  "WhlCmb"

== system Ebike_Thermal_DT_v1/Environment/Ground Feedback/3D Terrain/3D Engine Source/Single Point ==
  Bus Creator1 : BusCreator  Inputs=4
  Bus Selector2 : BusSelector  OutputSignals=Wheel1Positions,Wheel2Positions,Wheel3Positions,Wheel4Positions
  Constant2 : Constant  Value=repmat(eye(3),1,1,4)  SampleTime=-1
  Data Type Conversion{1..4} (4 alike) : DataTypeConversion  SaturateOnIntegerOverflow=off  RndMeth=Floor
  First Order Hold{5..8} (4 alike) : FirstOrderHold  ErrorTolerance=1
  Range Limiter{5..8} (4 alike) : Saturate  UpperLimit=1e3  LowerLimit=-1e3  ZeroCross=off
  Signal Specification{6..9} (4 alike) : SignalSpecification  Unit=m
  Simulation 3D Terrain Sensor1 : sim3dgroundtruthsensorlib/Simulation 3D Terrain Sensor  Priority=1  vehTagList={'Scene Origin';'SimulinkVehicle1'}  sensorTag=Sim3dSensor�  sensorId=1  sensorName=Sim3dSensor1  vehTag=SimulinkVehicle1  CoordinateSystem=Default  tmountOffset=[0, 0, 0]  rmountOffset=[0,0,0,]  RayOrigins=[0 0 1]  RayDirections=[0 0 -1]  RayLengths=20  NumberOfWheels=4  VisualizeTraceLines=off  SampleTime=-1  aMode=2  ID=1
  Zend Select{1..4} (4 alike) : Selector  NumberOfDimensions=2  InputPortWidth=3  IndexOptions=Select all,Index vector (dialog)  Indices=[1 3],3  OutputSizes=1,1
  z : Outport
  DCM : Outport  Port=2
  wires:
  Signal Specification6/1 -> Bus Creator1/1  "G_FL_z"
  Simulation 3D Terrain Sensor1/1 -> Bus Selector2/1
  Bus Selector2/4 -> Range Limiter8/1  "<Wheel4Positions>"
  Zend Select1/1 -> Data Type Conversion1/1
  Signal Specification7/1 -> Bus Creator1/2  "G_FR_z"
  Bus Selector2/2 -> Range Limiter6/1  "<Wheel2Positions>"
  Data Type Conversion3/1 -> First Order Hold7/1
  Data Type Conversion4/1 -> First Order Hold8/1
  Zend Select3/1 -> Data Type Conversion3/1
  First Order Hold6/1 -> Signal Specification7/1
  Zend Select2/1 -> Data Type Conversion2/1
  Data Type Conversion2/1 -> First Order Hold6/1
  Range Limiter6/1 -> Zend Select2/1
  Data Type Conversion1/1 -> First Order Hold5/1
  First Order Hold7/1 -> Signal Specification8/1
  Zend Select4/1 -> Data Type Conversion4/1
  Range Limiter8/1 -> Zend Select4/1
  Bus Selector2/1 -> Range Limiter5/1  "<Wheel1Positions>"
  First Order Hold8/1 -> Signal Specification9/1
  Bus Selector2/3 -> Range Limiter7/1  "<Wheel3Positions>"
  Range Limiter7/1 -> Zend Select3/1
  First Order Hold5/1 -> Signal Specification6/1
  Range Limiter5/1 -> Zend Select1/1
  Signal Specification8/1 -> Bus Creator1/3  "G_RL_z"
  Signal Specification9/1 -> Bus Creator1/4  "G_RR_z"
  Bus Creator1/1 -> z/1  "z"
  Constant2/1 -> DCM/1  "DCM"

== system Ebike_Thermal_DT_v1/Environment/Ground Feedback/Inclined Plane/Ideal Inclined Plane/Enabled ==
  Z : Inport
  phi : Inport  Port=2
  theta : Inport  Port=3
  Disabled : Subsystem  VariantControl=plane3D==0
  Enabled : Subsystem  VariantControl=plane3D==1

== system Ebike_Thermal_DT_v1/Environment/Varying Friction/Varying Friction/Road Track Friction/2D Lookup Tbl for Scaling Fctr (Lambda) ==
  XWhl : Inport  Partition=on  PartitionDimension=1  PartitionWidth=1  PartitionOffset=0
  YWhl : Inport  Port=2  Partition=on  PartitionDimension=1  PartitionWidth=1  PartitionOffset=0
  XBpt : Inport  Port=3
  YBpt : Inport  Port=4
  2-D Lookup Table : Lookup_n-D  BreakpointsForDimension1Source=Input port  BreakpointsForDimension1=xbr  BreakpointsForDimension2Source=Input port  BreakpointsForDimension2=ybr  Table=mutable  ExtrapMethod=Clip  InternalRulePriority=Speed  RndMeth=Simplest
      settings: InputPortMap=u0,u1,p5,p7
  For Each : ForEach  DisableCoverage=on
  Lambda for each whl : Outport  ConcatenationDimension=1
  wires:
  XWhl/1 -> 2-D Lookup Table/1
  YWhl/1 -> 2-D Lookup Table/2
  2-D Lookup Table/1 -> Lambda for each whl/1
  XBpt/1 -> 2-D Lookup Table/3
  YBpt/1 -> 2-D Lookup Table/4

== system Ebike_Thermal_DT_v1/Environment/Varying Friction/Varying Friction/Road Track Friction/Creating Inertial Frm Bpt ==
  XCg : Inport
  YCg : Inport  Port=2
  Enable : EnablePort
  Add : Sum
  Add1 : Sum
  Constant1 : Constant  Value=ybr
  Constant3 : Constant  Value=xbr
  XBpt : Outport
  YBpt : Outport  Port=2
  wires:
  Add/1 -> XBpt/1
  Constant1/1 -> Add1/1
  Add1/1 -> YBpt/1
  Constant3/1 -> Add/2
  YCg/1 -> Add1/2
  XCg/1 -> Add/1

== system Ebike_Thermal_DT_v1/Environment/Varying Friction/Varying Friction/Road Track Friction/En at t = 0 ==
  Clock1 : Clock
  Compare To Zero : simulink/Logic and Bit Operations/Compare To Zero  relop===  OutDataTypeStr=boolean
  Constant : Constant
  Constant2 : Constant  Value=0
  Switch1 : Switch  Criteria=u2 > Threshold  SaturateOnIntegerOverflow=off  InputSameDT=off
  Out1 : Outport
  wires:
  Clock1/1 -> Compare To Zero/1
  Constant2/1 -> Switch1/3
  Constant/1 -> Switch1/1
  Switch1/1 -> Out1/1
  Compare To Zero/1 -> Switch1/2

== system Ebike_Thermal_DT_v1/Environment/Ground Feedback/3D Terrain/3D Engine Source/Multiple Points/For Each Subsystem ==
  phi,theta,psi : Inport  Partition=on  PartitionDimension=2  PartitionWidth=1  PartitionOffset=0
  For Each : ForEach  DisableCoverage=on
  Rotation Angles to Direction Cosine Matrix1 : sharedtransform/Rotation Angles to Direction Cosine Matrix  rotationOrder=YXZ  aMode=2
  Selector5 : Selector  InputPortWidth=3  IndexOptions=Index vector (dialog)  Indices=[2 1 3]  OutputSizes=1
  WheelDCM : Outport  ConcatenationDimension=3
  wires:
  Selector5/1 -> Rotation Angles to Direction Cosine Matrix1/1
  Rotation Angles to Direction Cosine Matrix1/1 -> WheelDCM/1
  phi,theta,psi/1 -> Selector5/1

== system Ebike_Thermal_DT_v1/Environment/Ground Feedback/Inclined Plane/Ideal Inclined Plane/Enabled/Disabled ==

== system Ebike_Thermal_DT_v1/Environment/Ground Feedback/Inclined Plane/Ideal Inclined Plane/Enabled/Enabled ==
  Z : Inport
  phi : Inport  Port=2
  theta : Inport  Port=3
  Constant1 : Constant  Value=[planeX, planeY, 1]
  Constant4 : Constant  Value=0
  Constant5 : Constant  Value=0
  Mux : Mux  Inputs=3
  Mux1 : Mux  Inputs=3
  Reshape : Reshape  OutputDimensionality=Row vector (2-D)
  Reshape1 : Reshape  OutputDimensionality=Row vector (2-D)
  Reshape2 : Reshape  OutputDimensionality=Row vector (2-D)
  Signal Specification2 : SignalSpecification  Unit=deg
  Signal Specification3 : SignalSpecification  Unit=rad
  Simulation 3D Actor : sim3dlib/Simulation 3D Actor  Priority=1  ActorName=Plane  ParentName=Scene Origin  Operation=Create at setup  InitScriptText=|  SampleTime=-1  Translation=[0 0 Z_o]  Rotation=[phi_o theta_o 0]  Scale=[planeX planeY 1]  InputsText=|  aMode=5  ActorTag=Plane  ActorType=Sim3dActor  ID=C
      InitScriptText=|
      | planeSurface = sim3d.Actor('ActorName','BaseSurface');
      | Actor.propagate('CoordinateSystem',"ISO8855");
      | planeSurface.createShape('checker',[200,200,+0.03],[50,50]);
      | planeSurface.Translation = [0 0 0]; 
      | planeSurface.Shininess = 0;
      | planeSurface.Transparency = 0;
      | planeSurface.TextureMapping.Blend = 1;
      | planeSurface.TextureMapping.Roughness = .8;
      | World.add(planeSurface,Actor);
      InputsText=|
      | Plane.Translation
      | Plane.Rotation   
      | Plane.Scale
  Subtract : Sum  Inputs=+-
  Terminator : Terminator
  Unit Conversion1 : UnitConversion
  half plane thickness : Constant  Value=.015
  wires:
  Simulation 3D Actor/1 -> Terminator/1
  phi/1 -> Mux/1
  Constant5/1 -> Mux/3
  Reshape1/1 -> Simulation 3D Actor/2
  Constant4/1 -> Mux1/2, Mux1/1
  Reshape/1 -> Simulation 3D Actor/1
  Signal Specification2/1 -> Reshape1/1
  Reshape2/1 -> Simulation 3D Actor/3
  Constant1/1 -> Reshape2/1
  Z/1 -> Subtract/1
  Mux1/1 -> Reshape/1
  Subtract/1 -> Mux1/3
  half plane thickness/1 -> Subtract/2
  Unit Conversion1/1 -> Signal Specification2/1
  theta/1 -> Mux/2
  Signal Specification3/1 -> Unit Conversion1/1
  Mux/1 -> Signal Specification3/1

== matlab function Ebike_Thermal_DT_v1/Environment/Ground Feedback/Height Map/MATLAB Function ==
  data: grade input; DCMbe output
function DCMbe = pitchDCM(grade)
%#codegen

% Copyright 2025 The MathWorks, Inc.

% pitchDCM Generate body-to-earth DCM for ZYX order with only grade input
%   grade: scalar angle [rad]
%   DCM, rotation from body to earth
    cp = cos(grade);
    sp = sin(grade);
    DCMbe = [ cp,  0,  sp;
           0,  1,   0;
         -sp,  0,  cp ];
end

== matlab function Ebike_Thermal_DT_v1/Environment/Ground Feedback/Inclined Plane/Ideal Inclined Plane/Z Plane ==
  data: X input; Z output; Y input; Zoffset input; phi input; theta input; DCM output
function [Z,DCM] = Zplane(X,Y,Zoffset,phi,theta)%#codege
 coder.allowpcode('plain')
 [Z,DCM] = vdynblksZplane(X,Y,Zoffset,phi,theta);
end

== matlab function Ebike_Thermal_DT_v1/Environment/Ground Feedback/Constant/MATLAB Function ==
  data: grade input; DCMbe output
function DCMbe = pitchDCM(grade)
%#codegen

% Copyright 2025 The MathWorks, Inc.

% pitchDCM Generate body-to-earth DCM for ZYX order with only grade input
%   grade: scalar angle [rad]
%   DCM, rotation from body to earth
    cp = cos(grade);
    sp = sin(grade);
    DCMbe = [ cp,  0,  sp;
           0,  1,   0;
         -sp,  0,  cp ];
end

== matlab function Ebike_Thermal_DT_v1/Environment/Subsystem/Estimated Grade ==
  data: DCMs input; Grade output
function Grade = DCM2Grade(DCMs)
%#codegen
% use the world to body DCM to extract the estimated pitch angle (grade)
N = size(DCMs, 3);
thetas = zeros(N,1);
for idx = 1:N
    DCM = DCMs(:,:,idx);
    thetas(idx) = asin(DCM(1,3));  % For world-to-body, ZYX
end
Grade =  mean(thetas)*180/pi;
end
